simulink model "spaceship_temp"  (R2023b)
settings: Solver=ode45  StartTime=0.0  StopTime=30  RelTol=1e-3  EnableMultiTasking=on
libraries: vrlib x2, sharedtransform x1, simulink_extras x1
Description:
  | Plane Take-Off with HUD Text
  | 
  | This model is a variant of the vrtkoff example that shows also how to display
  | signal values as text in the virtual scene and a simple Head-Up Display (HUD).
  | 
  | The text is sent to the virtual world as Simulink(R) string signal, composed from the numeric
  | input values using the format string (see sprintf for more information) and sent
  | to the 'string' field of the corresponding Text node in the world. Individual lines of
  | the MFString field are separated by the newline character in the format string.
  | 
  | The HUD behavior (maintaining constant relative position between the user and the
  | Text node) is achieved by defining a ProximitySensor that senses user position and
  | orientation as it navigates through the scene and routing this information to the translation
  | and rotation of HUD object - in this case a VRML Transform that contains the Text node.
settings Model: Creator=The MathWorks, Inc.  LastModifiedBy=therkelsen
settings SolverCC: AlgebraicLoopSolver=TrustRegion
settings DataIOCC: LimitDataPoints=on  SaveFormat=Array  SaveOutput=off  SaveTime=off  ReturnWorkspaceOutputs=off  SignalLoggingName=logsOut
settings OptimizationCC: BlockReduction=off  BooleanDataType=off  ExpressionDepthLimit=2147483647  InitFltsAndDblsToZero=on  LifeSpan=inf
settings DebuggingCC: UnderspecifiedInitializationDetection=Classic  MergeDetectMultiDrivingBlocksExec=none  CheckExecutionContextPreStartOutputMsg=on  SignalResolutionControl=TryResolveAllWithWarning  MultiTaskDSMMsg=warning  MultiTaskCondExecSysMsg=none  FcnCallInpInsideContextMsg=warning  UnconnectedInputMsg=warning  UnconnectedOutputMsg=warning  UnconnectedLineMsg=warning  StateNameClashWarn=warning  SymbolicDimsDataTypeCodeGenerationDiagnostic=none  SFUnexpectedBacktrackingDiag=warning  SFNoUnconditionalDefaultTransitionDiag=warning  SFExecutionAtInitializationDiag=none  ArithmeticOperatorsInVariantConditions=warning
settings HardwareCC: ProdBitPerPointer=32  ProdBitPerSizeT=32  ProdBitPerPtrDiffT=32  ProdLargestAtomicFloat=None  ProdIntDivRoundTo=Undefined  ProdEndianess=Unspecified  ProdWordSize=32  ProdHWDeviceType=32-bit Generic  TargetUnknown=on
settings ModelReferenceCC: UpdateModelReferenceTargets=IfOutOfDate  EnableRefExpFcnMdlSchedulingChecks=on  PropagateSignalLabelsOutOfModel=off
settings SFSimCC: SimUseLocalCustomCode=off  CustomCodeUndefinedFunction=UseInterfaceOnly
settings RTWCC: RTWUseLocalCustomCode=off  DLArmComputeVersion=19.05
settings CodeAppCC: StateflowObjectComments=on
settings GRTTargetCC: TargetFcnLib=ansi_tfl_tmw.mat  TargetLangStandard=C89/C90 (ANSI)  CombineOutputUpdateFcns=off  GRTInterface=on
settings ConfigComp: CovMetricSettings=d  CovSaveCumulativeToWorkspaceVar=on  CovSaveSingleToWorkspaceVar=on  CovExternalEMLEnable=off  CovSFcnEnable=off

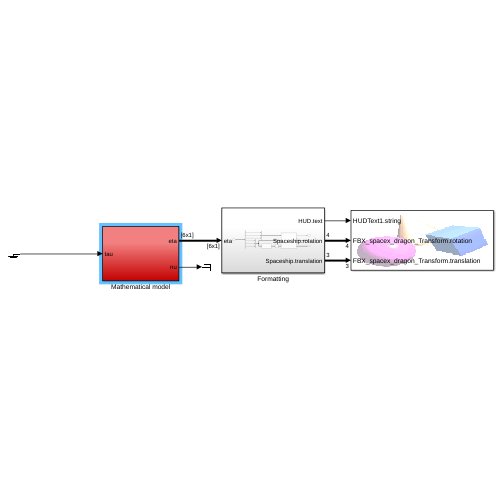
[thumbnail: Simulink's stored preview of the top-level diagram]
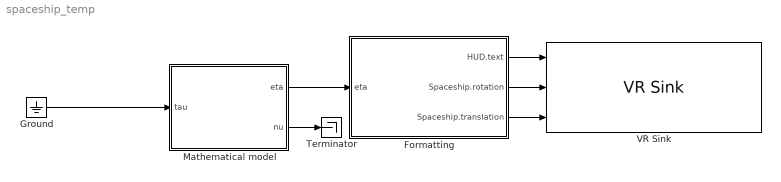
== system spaceship_temp ==
  Formatting : Subsystem
  Ground : Ground
  Mathematical model : Subsystem
  Terminator : Terminator
  VR Sink : vrlib/VR Sink  InstantiateOnLoad=on  SampleTime=0.1  ViewEnable=on  RemoteChange=off  RemoteView=off  FieldsWritten=HUDText1.string.1.-1.1.char#FBX_spacex_dragon_Transform.rotation.4.1.1.double#FBX_spacex_dragon_Transform.translation.3.1.1.double  WorldFileName=spaceship_VR.x3d  WorldDescription=VR Spaceship Dragon  AutoView=off  VideoDimensions=[]  AllowVariableSize=off
  wires:
  Formatting/1(HUD.text) -> VR Sink/1
  Formatting/2(Spaceship.rotation) -> VR Sink/2
  Formatting/3(Spaceship.translation) -> VR Sink/3
  Mathematical model/1(eta) -> Formatting/1(eta)
  Mathematical model/2(nu) -> Terminator/1
  Ground/1 -> Mathematical model/1(tau)

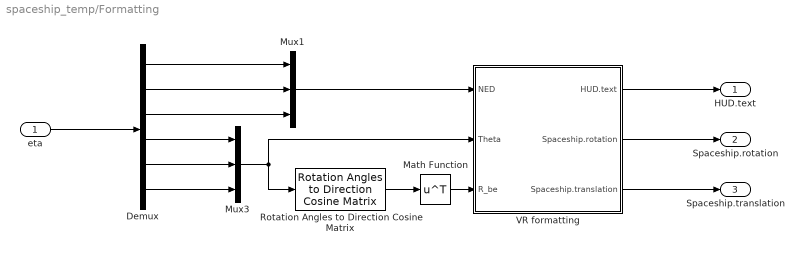
== system spaceship_temp/Formatting ==
  eta : Inport
  Demux : Demux  Outputs=6
  Math Function : Math  Operator=transpose
  Mux1 : Mux  Inputs=3
  Mux3 : Mux  Inputs=3
  Rotation Angles to Direction Cosine Matrix : sharedtransform/Rotation Angles to Direction Cosine Matrix  rotationOrder=XYZ  aMode=aMode
  VR formatting : Subsystem
  HUD.text : Outport
  Spaceship.rotation : Outport  Port=2
  Spaceship.translation : Outport  Port=3
  wires:
  Demux/2 -> Mux1/2
  Demux/3 -> Mux1/3
  Mux1/1 -> VR formatting/1(NED)
  Demux/5 -> Mux3/2
  eta/1 -> Demux/1
  Demux/4 -> Mux3/1
  Demux/6 -> Mux3/3
  Math Function/1 -> VR formatting/3(R_be)
  Rotation Angles to Direction Cosine Matrix/1 -> Math Function/1
  Demux/1 -> Mux1/1
  VR formatting/1(HUD.text) -> HUD.text/1
  VR formatting/2(Spaceship.rotation) -> Spaceship.rotation/1
  VR formatting/3(Spaceship.translation) -> Spaceship.translation/1
  Mux3/1 -> Rotation Angles to Direction Cosine Matrix/1, VR formatting/2(Theta)

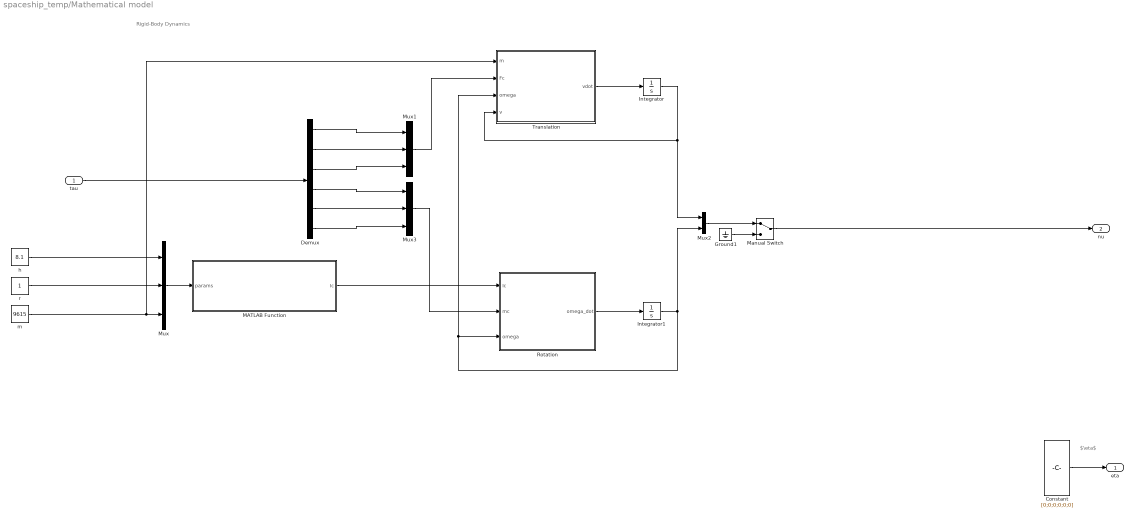
== system spaceship_temp/Mathematical model ==
  note: Rigid-Body Dynamics
  note: $\eta$
  tau : Inport
  Constant : Constant  Value=[0;0;0;0;0;0]  VectorParams1D=off
  Demux : Demux  Outputs=6
  Ground1 : Ground
  Integrator : Integrator  InitialCondition=[1,1,1]
  Integrator1 : Integrator  InitialCondition=[1,1,1]
  MATLAB Function : MATLAB Function  TreatAsAtomicUnit=on
  Manual Switch : ManualSwitch
  Mux : Mux  Inputs=3
  Mux1 : Mux  Inputs=3
  Mux2 : Mux  Inputs=2
  Mux3 : Mux  Inputs=3
  Rotation : MATLAB Function  TreatAsAtomicUnit=on
  Translation : MATLAB Function  TreatAsAtomicUnit=on
  h : Constant  Value=8.1
  m : Constant  Value=9615
  r : Constant
  eta : Outport
  nu : Outport  Port=2
  wires:
  Constant/1 -> eta/1
  Ground1/1 -> Manual Switch/2
  Manual Switch/1 -> nu/1
  Mux2/1 -> Manual Switch/1
  Mux1/1 -> Translation/2(Fc)
  Integrator/1 -> Translation/4(v), Mux2/1
  r/1 -> Mux/2
  Demux/6 -> Mux3/3
  Integrator1/1 -> Translation/3(omega), Rotation/3(omega), Mux2/2
  Demux/4 -> Mux3/1
  Mux/1 -> MATLAB Function/1(params)
  Demux/5 -> Mux3/2
  MATLAB Function/1(Ic) -> Rotation/1(Ic)
  tau/1 -> Demux/1
  Demux/3 -> Mux1/3
  Rotation/1(omega_dot) -> Integrator1/1
  m/1 -> Mux/3, Translation/1(m)
  h/1 -> Mux/1
  Demux/1 -> Mux1/1
  Demux/2 -> Mux1/2
  Translation/1(vdot) -> Integrator/1
  Mux3/1 -> Rotation/2(mc)

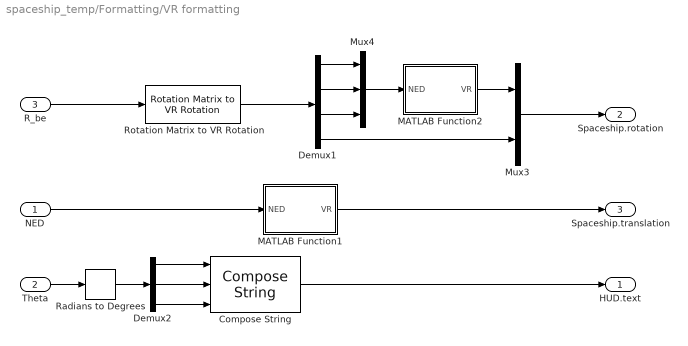
== system spaceship_temp/Formatting/VR formatting ==
  NED : Inport
  Theta : Inport  Port=2
  R_be : Inport  Port=3
  Compose String : ComposeString  Format="'Roll    : %7.2f deg\\nPitch   : %7.2f deg\\nYaw     : %7.2f deg'"
  Demux1 : Demux
  Demux2 : Demux  Outputs=3
  MATLAB Function1 : MATLAB Function  TreatAsAtomicUnit=on
  MATLAB Function2 : MATLAB Function  TreatAsAtomicUnit=on
  Mux3 : Mux  Inputs=2
  Mux4 : Mux  Inputs=3
  Radians to Degrees : simulink_extras/Transformations/Radians to Degrees
  Rotation Matrix to VR Rotation : vrlib/Utilities/Rotation Matrix to VR Rotation  maxzero=1e-12
  HUD.text : Outport
  Spaceship.rotation : Outport  Port=2
  Spaceship.translation : Outport  Port=3
  wires:
  Rotation Matrix to VR Rotation/1 -> Demux1/1
  Mux3/1 -> Spaceship.rotation/1
  MATLAB Function2/1(VR) -> Mux3/1
  Mux4/1 -> MATLAB Function2/1(NED)
  Demux1/3 -> Mux4/3
  Demux1/1 -> Mux4/1
  Demux1/2 -> Mux4/2
  Demux1/4 -> Mux3/2
  NED/1 -> MATLAB Function1/1(NED)
  MATLAB Function1/1(VR) -> Spaceship.translation/1
  Demux2/1 -> Compose String/1
  Demux2/2 -> Compose String/2
  Demux2/3 -> Compose String/3
  Compose String/1 -> HUD.text/1
  Theta/1 -> Radians to Degrees/1
  R_be/1 -> Rotation Matrix to VR Rotation/1
  Radians to Degrees/1 -> Demux2/1

== matlab function spaceship_temp/Mathematical model/Rotation ==
  data: Ic input; omega_dot output; mc input; omega input
function omega_dot = rotational_motion(Ic, mc, omega)

omega_dot = inv(Ic)*(mc - cross(omega, Ic*omega));

== matlab function spaceship_temp/Mathematical model/MATLAB Function ==
  data: params input; Ic output
function Ic = cylinder_inertia_tensor(params)

h = params(1)
r = params(2)
m = params(3)

Ic = [1/12*m*(3*r^2 + h^2) 0 0;
               0 1/12*m*(3*r^2 + h^2) 0;
               0 0 1/2*m*r^2];

== matlab function spaceship_temp/Mathematical model/Translation ==
  data: m input; vdot output; Fc input; omega input; v input
function vdot = translational_motion(m, Fc, omega, v)

vdot = 1/m * (Fc - cross(omega, m*v));

== matlab function spaceship_temp/Formatting/VR formatting/MATLAB Function1 ==
  data: NED input; VR output
function VR = NED2VR(NED)

x = NED(1); % north
y = NED(2); % east 
z = NED(3); % down

VR = [ -y ; -z ; x ];

== matlab function spaceship_temp/Formatting/VR formatting/MATLAB Function2 ==
  data: NED input; VR output
function VR = NED2VR(NED)

x = NED(1); % north
y = NED(2); % east 
z = NED(3); % down

VR = [ -y ; -z ; x ];
